simulink model "pid_demo"  (R2020a)
settings: Solver=VariableStepAuto  StartTime=0.0  StopTime=40  RelTol=1e-3
values from neighbouring files (symbols this model uses):
  aubr = -8:0.05:5    [generate_calibration.m]
  tablebr = zeros(length(vubr),length(aubr))    [generate_calibration.m]
  vubr = 0:0.05:50    [generate_calibration.m]
  x = x-0.1    (= -0.1)    [brake_calibration.m]    (also in thr_calibration.m = 0.05)
libraries: simulink x2, Solver_SF x1
settings Model: Creator=wwcong  LastModifiedBy=czj
settings DataIOCC: ReturnWorkspaceOutputs=off
settings DebuggingCC: ArithmeticOperatorsInVariantConditions=warning
settings SFSimCC: SimUseLocalCustomCode=off  CustomCodeUndefinedFunction=UseInterfaceOnly
settings RTWCC: RTWUseLocalCustomCode=off

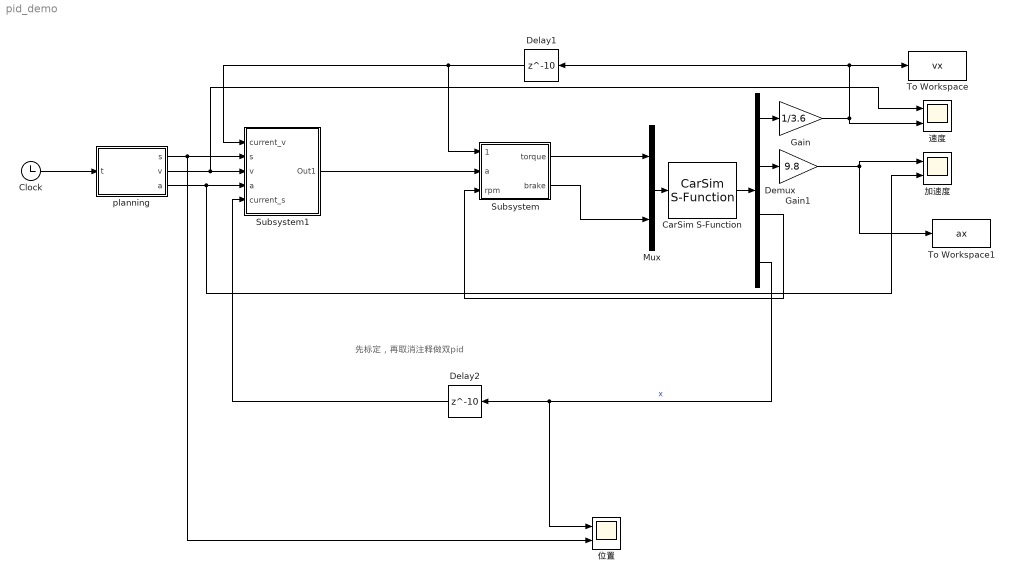
== system pid_demo ==
  note: 先标定，再取消注释做双pid
  CarSim S-Function : Solver_SF/CarSim S-Function  Priority=1  SIMFILE=simfile.sim  Run_RTs=off  vs_state_ind=Run  StopMode_ind=Vehicle Model
  Clock : Clock
  Delay1 : Delay  DelayLength=10
  Delay2 : Delay  DelayLength=10
  Demux : Demux
  Gain : Gain  Gain=1/3.6
  Gain1 : Gain  Gain=9.8
  Mux : Mux  Inputs=2
  Subsystem : Subsystem
  Subsystem1 : Subsystem
  To Workspace : ToWorkspace  VariableName=vx  SaveFormat=Timeseries  SampleTime=0.1
  To Workspace1 : ToWorkspace  VariableName=ax  SaveFormat=Timeseries  SampleTime=0.1
  planning : MATLAB Function  TreatAsAtomicUnit=on
  位置 : Scope  NumInputPorts=2
  加速度 : Scope  NumInputPorts=2
  速度 : Scope  NumInputPorts=2
  wires:
  Mux/1 -> CarSim S-Function/1
  CarSim S-Function/1 -> Demux/1
  Demux/1 -> Gain/1
  Demux/2 -> Gain1/1
  Gain1/1 -> To Workspace1/1, 加速度/1
  Gain/1 -> 速度/2, Delay1/1, To Workspace/1
  Clock/1 -> planning/1(t)
  Demux/3 -> Subsystem/3(rpm)
  Subsystem/1(torque) -> Mux/1
  Subsystem/2(brake) -> Mux/2
  Delay1/1 -> Subsystem1/1(current_v), Subsystem/1(current_v)
  Demux/4 -> 位置/1, Delay2/1  "x"
  planning/1(s) -> 位置/2, Subsystem1/2(s)
  planning/2(v) -> 速度/1, Subsystem1/3(v)
  planning/3(a) -> 加速度/2, Subsystem1/4(a)
  Delay2/1 -> Subsystem1/5(current_s)
  Subsystem1/1(Out1) -> Subsystem/2(a)

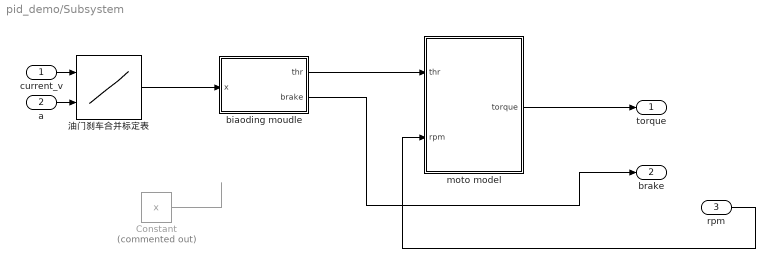
== system pid_demo/Subsystem ==
  current_v : Inport
  a : Inport  Port=2
  rpm : Inport  Port=3
  Constant : Constant  Commented=on  Value=x
  biaoding moudle : MATLAB Function  TreatAsAtomicUnit=on
  moto model : MATLAB Function  TreatAsAtomicUnit=on
  油门刹车合并标定表 : Lookup_n-D  BreakpointsForDimension1=vubr  BreakpointsForDimension2=aubr  Table=tablebr  InternalRulePriority=Speed  RndMeth=Simplest  InputSameDT=on
  torque : Outport
  brake : Outport  Port=2
  wires:
  biaoding moudle/2(brake) -> brake/1
  moto model/1(torque) -> torque/1
  biaoding moudle/1(thr) -> moto model/1(thr)
  rpm/1 -> moto model/2(rpm)
  a/1 -> 油门刹车合并标定表/2
  current_v/1 -> 油门刹车合并标定表/1
  油门刹车合并标定表/1 -> biaoding moudle/1(x)
  Constant/1 -> ?

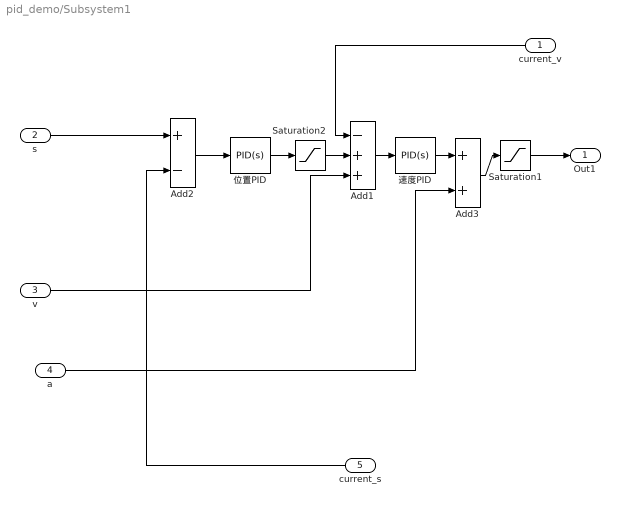
== system pid_demo/Subsystem1 ==
  current_v : Inport
  s : Inport  Port=2
  v : Inport  Port=3
  a : Inport  Port=4
  current_s : Inport  Port=5
  Add1 : Sum  Inputs=-++
  Add2 : Sum  Inputs=+-
  Add3 : Sum
  Saturation1 : Saturate  UpperLimit=5  LowerLimit=-8
  Saturation2 : Saturate  UpperLimit=10  LowerLimit=-10
  位置PID : simulink/Continuous/PID Controller  Controller=PID  Form=Parallel  TimeDomain=Continuous-time  UseExternalTs=off  SampleTime=-1  IntegratorMethod=Forward Euler  FilterMethod=Forward Euler  ControllerParametersSource=internal  P=3  I=0.01  D=0.1  UseFilter=on  N=30  TunerSelectOption=Transfer Function Based (PID Tuner App)  InitialConditionSource=internal  InitialConditionForIntegrator=0  InitialConditionForFilter=0  DifferentiatorICPrevScaledInput=0  ExternalReset=none  TrackingMode=off  Kt=1  LimitOutput=off  UpperSaturationLimit=inf  LowerSaturationLimit=-inf  LinearizeAsGain=on  AntiWindupMode=none  Kb=1  POutMin=[]  POutMax=[]  IOutMin=[]  IOutMax=[]  DOutMin=[]  DOutMax=[]  NOutMin=[]  NOutMax=[]  SumOutMin=[]  SumOutMax=[]  SaturationOutMin=[]  SaturationOutMax=[]  PParamMin=[]  PParamMax=[]  IParamMin=[]  IParamMax=[]  DParamMin=[]  DParamMax=[]  NParamMin=[]  NParamMax=[]  KbParamMin=[]  KbParamMax=[]  KtParamMin=[]  KtParamMax=[]  KbOutMin=[]  KbOutMax=[]  KtOutMin=[]  KtOutMax=[]  IntegratorOutMin=[]  IntegratorOutMax=[]  FilterOutMin=[]  FilterOutMax=[]  SumI1OutMin=[]  SumI1OutMax=[]  SumI2OutMin=[]  SumI2OutMax=[]  SumI3OutMin=[]  SumI3OutMax=[]  SumI4OutMin=[]  SumI4OutMax=[]  SumDOutMin=[]  SumDOutMax=[]  DifferentiatorOutMin=[]  DifferentiatorOutMax=[]  FilterDiffOutCoefMin=[]  FilterDiffOutCoefMax=[]  ReciprocalOutMin=[]  ReciprocalOutMax=[]  SumDenOutMin=[]  SumDenOutMax=[]  SumNumOutMin=[]  SumNumOutMax=[]  DivideOutMin=[]  DivideOutMax=[]  UdiffTsProdOutMin=[]  UdiffTsProdOutMax=[]  NTsProdOutMin=[]  NTsProdOutMax=[]  UintegralTsProdOutMin=[]  UintegralTsProdOutMax=[]  UngainTsProdOutMin=[]  UngainTsProdOutMax=[]  IntegratorContinuousStateAttributes=''  IntegratorStateMustResolveToSignalObject=off  IntegratorRTWStateStorageClass=Auto  FilterContinuousStateAttributes=''  FilterStateMustResolveToSignalObject=off  FilterRTWStateStorageClass=Auto  ParallelPVariant=InternalParameters  IdealPVariant=Disabled  IVariant=InternalParameters  DVariant=InternalParameters  IntegratorVariant=Continuous  SatVariant=Disabled  AWVariant=Passthrough  PCopyVariant=Disabled  TRVariant=Disabled  FdbkBlocksVariant=Forward  IdealPFdbkVariant=Disabled  SatFdbkVariant=Disabled  DerivativeFilterVariant=ContFilter  NVariant=InternalParameters  NCopyVariant=Disabled  FilterICVariant=InternalICsFilter  IntegratorICVariant=InternalICs  ExternalResetVariant=Disabled  TRSumVariant=Passthrough  SumFdbkVariant=Disabled  SumVariant=Sum_PID  TsampFilterVariant=InternalTs  TsampNgainVariant=Passthrough  TsampIntegralVariant=Passthrough
  速度PID : simulink/Continuous/PID Controller  Controller=PID  Form=Parallel  TimeDomain=Continuous-time  UseExternalTs=off  SampleTime=-1  IntegratorMethod=Forward Euler  FilterMethod=Forward Euler  ControllerParametersSource=internal  P=3  I=0.001  D=2  UseFilter=on  N=30  TunerSelectOption=Transfer Function Based (PID Tuner App)  InitialConditionSource=internal  InitialConditionForIntegrator=0  InitialConditionForFilter=0  DifferentiatorICPrevScaledInput=0  ExternalReset=none  TrackingMode=off  Kt=1  LimitOutput=off  UpperSaturationLimit=inf  LowerSaturationLimit=-inf  LinearizeAsGain=on  AntiWindupMode=none  Kb=1  POutMin=[]  POutMax=[]  IOutMin=[]  IOutMax=[]  DOutMin=[]  DOutMax=[]  NOutMin=[]  NOutMax=[]  SumOutMin=[]  SumOutMax=[]  SaturationOutMin=[]  SaturationOutMax=[]  PParamMin=[]  PParamMax=[]  IParamMin=[]  IParamMax=[]  DParamMin=[]  DParamMax=[]  NParamMin=[]  NParamMax=[]  KbParamMin=[]  KbParamMax=[]  KtParamMin=[]  KtParamMax=[]  KbOutMin=[]  KbOutMax=[]  KtOutMin=[]  KtOutMax=[]  IntegratorOutMin=[]  IntegratorOutMax=[]  FilterOutMin=[]  FilterOutMax=[]  SumI1OutMin=[]  SumI1OutMax=[]  SumI2OutMin=[]  SumI2OutMax=[]  SumI3OutMin=[]  SumI3OutMax=[]  SumI4OutMin=[]  SumI4OutMax=[]  SumDOutMin=[]  SumDOutMax=[]  DifferentiatorOutMin=[]  DifferentiatorOutMax=[]  FilterDiffOutCoefMin=[]  FilterDiffOutCoefMax=[]  ReciprocalOutMin=[]  ReciprocalOutMax=[]  SumDenOutMin=[]  SumDenOutMax=[]  SumNumOutMin=[]  SumNumOutMax=[]  DivideOutMin=[]  DivideOutMax=[]  UdiffTsProdOutMin=[]  UdiffTsProdOutMax=[]  NTsProdOutMin=[]  NTsProdOutMax=[]  UintegralTsProdOutMin=[]  UintegralTsProdOutMax=[]  UngainTsProdOutMin=[]  UngainTsProdOutMax=[]  IntegratorContinuousStateAttributes=''  IntegratorStateMustResolveToSignalObject=off  IntegratorRTWStateStorageClass=Auto  FilterContinuousStateAttributes=''  FilterStateMustResolveToSignalObject=off  FilterRTWStateStorageClass=Auto  ParallelPVariant=InternalParameters  IdealPVariant=Disabled  IVariant=InternalParameters  DVariant=InternalParameters  IntegratorVariant=Continuous  SatVariant=Disabled  AWVariant=Passthrough  PCopyVariant=Disabled  TRVariant=Disabled  FdbkBlocksVariant=Forward  IdealPFdbkVariant=Disabled  SatFdbkVariant=Disabled  DerivativeFilterVariant=ContFilter  NVariant=InternalParameters  NCopyVariant=Disabled  FilterICVariant=InternalICsFilter  IntegratorICVariant=InternalICs  ExternalResetVariant=Disabled  TRSumVariant=Passthrough  SumFdbkVariant=Disabled  SumVariant=Sum_PID  TsampFilterVariant=InternalTs  TsampNgainVariant=Passthrough  TsampIntegralVariant=Passthrough
  Out1 : Outport
  wires:
  s/1 -> Add2/1
  Add1/1 -> 速度PID/1
  Add3/1 -> Saturation1/1
  Saturation1/1 -> Out1/1
  Add2/1 -> 位置PID/1
  位置PID/1 -> Saturation2/1
  速度PID/1 -> Add3/1
  current_s/1 -> Add2/2
  current_v/1 -> Add1/1
  Saturation2/1 -> Add1/2
  v/1 -> Add1/3
  a/1 -> Add3/2

== matlab function pid_demo/Subsystem/moto model ==
  data: thr input; torque output; rpm input
function torque = fcn(thr,rpm)
Tmax=380*thr;
    if (rpm<=4523)
        torque=Tmax;
    else
        torque=Tmax*4523/rpm;
    end
end

== matlab function pid_demo/planning ==
  data: t input; s output; v output; a output
function [s,v,a] = fcn(t)
if t<10
    s=0.1*t^3/3;
    v=0.1*t^2;
    a=0.2*t;
else
    a=2-0.1*(t-10);
    v=2*t-0.05*(t-10)^2-10;
    s=t^2-0.05*(t-10)^3/3-10*t+100/3;
end

== matlab function pid_demo/Subsystem/biaoding moudle ==
  data: x input; thr output; brake output
function [thr,brake] = fcn(x)
    %正数代表油门，负数代表刹车
    %不允许同时踩油门和刹车
    if x>=0
        thr=x;
        brake=0;
    else
        thr=0;
        brake=-x;
    end
